simulink model "MyElasticRobotJointSim"  (R2024b)
settings: Solver=VariableStepAuto  StartTime=0.0  StopTime=10  RelTol=1e-3
PostLoadFcn:
  | load
values from neighbouring files (symbols this model uses):
  K = 500    [FUNZIONA_CHISSA.m]    (also in identificazione_diagrammi_bode.m; robot_diverse_traiettorie.m = 2000; run_robot_simulation.m = 2000)
  M = 2    [FUNZIONA_CHISSA.m]    (also in identificazione_diagrammi_bode.m; robot_diverse_traiettorie.m; run_robot_simulation.m)
  Mm = 0.5    [FUNZIONA_CHISSA.m]    (also in identificazione_diagrammi_bode.m; robot_diverse_traiettorie.m; run_robot_simulation.m)
  Pg = 5    [robot_diverse_traiettorie.m]    (also in run_robot_simulation.m)
settings Model: Creator=riccardodaguanno  LastModifiedBy=riccardodaguanno

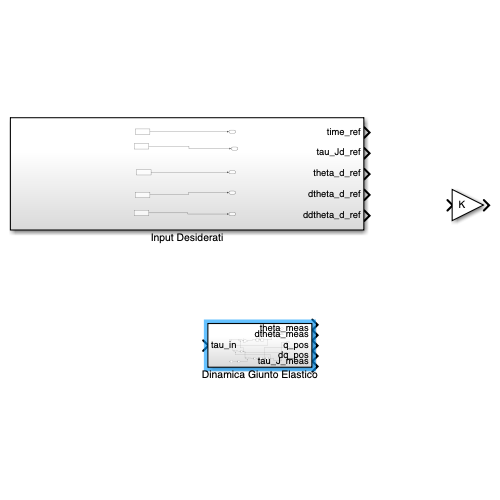
[thumbnail: Simulink's stored preview of the top-level diagram]
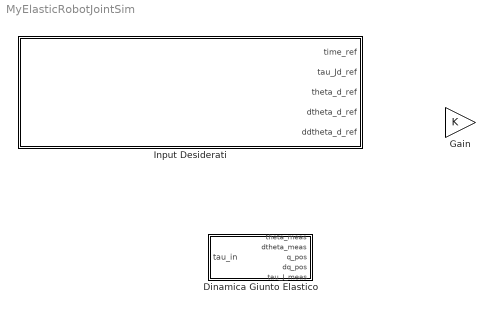
== system MyElasticRobotJointSim ==
  Dinamica Giunto Elastico : Subsystem
  Gain : Gain  Gain=K
  Input Desiderati : Subsystem

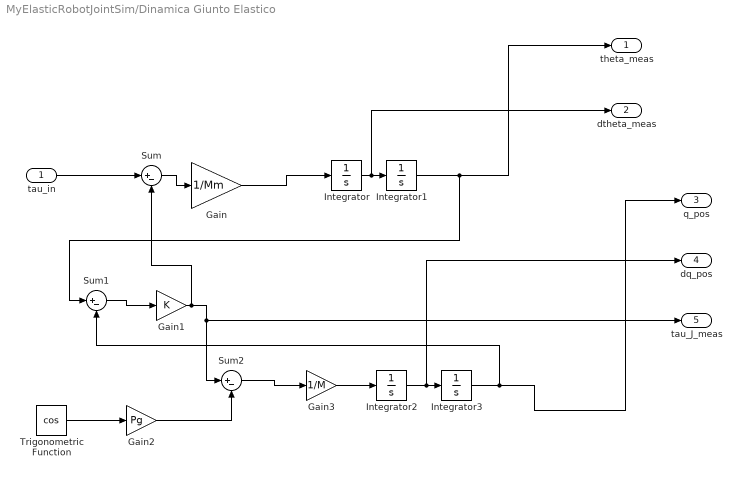
== system MyElasticRobotJointSim/Dinamica Giunto Elastico ==
  tau_in : Inport
  Gain : Gain  Gain=1/Mm
  Gain1 : Gain  Gain=K
  Gain2 : Gain  Gain=Pg
  Gain3 : Gain  Gain=1/M
  Integrator{,1..3} (4 alike) : Integrator
  Sum : Sum  Inputs=|+-
  Sum1 : Sum  Inputs=|+-
  Sum2 : Sum  Inputs=|+-
  Trigonometric Function : Trigonometry  Operator=cos
  theta_meas : Outport
  dtheta_meas : Outport  Port=2
  q_pos : Outport  Port=3
  dq_pos : Outport  Port=4
  tau_J_meas : Outport  Port=5
  wires:
  tau_in/1 -> Sum/1
  Sum/1 -> Gain/1
  Gain/1 -> Integrator/1
  Integrator/1 -> dtheta_meas/1, Integrator1/1
  Integrator1/1 -> Sum1/1, theta_meas/1
  Sum1/1 -> Gain1/1
  Gain1/1 -> Sum/2, tau_J_meas/1, Sum2/1
  Trigonometric Function/1 -> Gain2/1
  Gain2/1 -> Sum2/2
  Sum2/1 -> Gain3/1
  Gain3/1 -> Integrator2/1
  Integrator2/1 -> dq_pos/1, Integrator3/1
  Integrator3/1 -> Sum1/2, q_pos/1

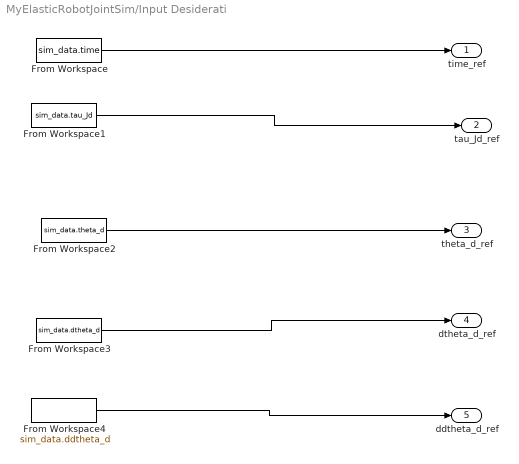
== system MyElasticRobotJointSim/Input Desiderati ==
  From Workspace : FromWorkspace  VariableName=sim_data.time
  From Workspace1 : FromWorkspace  VariableName=sim_data.tau_Jd
  From Workspace2 : FromWorkspace  VariableName=sim_data.theta_d
  From Workspace3 : FromWorkspace  VariableName=sim_data.dtheta_d
  From Workspace4 : FromWorkspace  VariableName=sim_data.ddtheta_d
  time_ref : Outport
  tau_Jd_ref : Outport  Port=2
  theta_d_ref : Outport  Port=3
  dtheta_d_ref : Outport  Port=4
  ddtheta_d_ref : Outport  Port=5
  wires:
  From Workspace4/1 -> ddtheta_d_ref/1
  From Workspace3/1 -> dtheta_d_ref/1
  From Workspace2/1 -> theta_d_ref/1
  From Workspace1/1 -> tau_Jd_ref/1
  From Workspace/1 -> time_ref/1
